simulink model "question2_c"  (R2019b)
settings: Solver=VariableStepAuto  StartTime=0.0  StopTime=10.0  RelTol=1e-3
libraries: fuzblock x50
(part 2 of 2)

== matlab function question2_c/lambda = 10/Subsystem/MATLAB Function ==
  data: A_2 input; y output; A_1 input; A0 input; A1 input; A2 input; B_2 input; B_1 input; B0 input; B1 input; B2 input
function y = fcn(A_2, A_1, A0, A1, A2, B_2, B_1, B0, B1, B2)
u_2_2 = -1;
u_2_1 = -0.7;
u_20 = -0.5;
u_21 = -0.3;
u_22 = 0;

u_1_2 = -0.7;
u_1_1 = -0.4;
u_10 = -0.2;
u_11 = 0;
u_12 = 0.3;

u0_2 = -0.5;
u0_1 = -0.2;
u00 = 0;
u01 = 0.2;
u02 = 0.5;

u1_2 = -0.3;
u1_1 = 0;
u10 = 0.2;
u11 = 0.4;
u12 = 0.7;

u2_2 = 0;
u2_1 = 0.3;
u20 = 0.5;
u21 = 0.7;
u22 = 1;

if ((A0==0) && (A1==0) && (A2==0)) % A_1 ve A_2
    
    if((B0==0) && (B1==0) && (B2==0) && (B_1~= 0) && (B_2~= 0))
        y = A_2*B_2*u_2_2 + A_2*B_1*u_2_1 + A_1*B_1*u_1_1 + A_1*B_2*u_1_2;
    
    elseif((B_2==0) && (B1==0) && (B2==0) && (B_1~= 0) && (B0~= 0))
        y = A_2*B_1*u_2_1 + A_2*B0*u_20 + A_1*B_1*u_1_1 + A_1*B0*u_10;
    
    elseif((B_2==0) && (B_1==0) && (B2==0) && (B0~= 0) && (B1~= 0))
        y = A_2*B0*u_20 + A_2*B1*u_21 + A_1*B0*u_10 + A_1*B1*u_11;
    
    elseif((B0==0) && (B_1==0) && (B_2==0) && (B1~= 0) && (B2~= 0))
        y = A_2*B1*u_21 + A_2*B2*u_22 + A_1*B1*u_11 + A_1*B2*u_12;
    
    elseif((B_1==0) && (B0==0) && (B1==0) && (B2==0))
        y = A_2*B_2*u_2_2 + A_1*B_2*u_1_2;
    
    elseif((B_2==0) && (B0==0) && (B1==0) && (B2==0))
        y = A_2*B_1*u_2_1 + A_1*B_1*u_1_1;
    
    elseif((B_2==0) && (B_1==0) && (B1==0) && (B2==0))
        y = A_2*B0*u_20 + A_1*B0*u_10;
    
    elseif((B_2==0) && (B_1==0) && (B0==0) && (B2==0))
        y = A_2*B1*u_21 + A_1*B1*u_11;
    
    elseif((B_2==0) && (B_1==0) && (B0==0) && (B1==0))
        y = A_2*B2*u_22 + A_1*B2*u_12;
    
    else
        y=0.5;
    end
    
elseif ((A_2==0) && (A1==0) && (A2==0)) % A_1 ve A0
    
    if((B0==0) && (B1==0) && (B2==0) && (B_1~= 0) && (B_2~= 0))
        y = A0*B_2*u0_2 + A0*B_1*u0_1 + A_1*B_1*u_1_1 + A_1*B_2*u_1_2;
    
    elseif((B_2==0) && (B1==0) && (B2==0) && (B_1~= 0) && (B0~= 0))
        y = A0*B_1*u0_1 + A0*B0*u00 + A_1*B_1*u_1_1 + A_1*B0*u_10;
    
    elseif((B_2==0) && (B_1==0) && (B2==0) && (B0~= 0) && (B1~= 0))
        y = A0*B0*u00 + A0*B1*u01 + A_1*B0*u_10 + A_1*B1*u_11;
    
    elseif((B0==0) && (B_1==0) && (B_2==0) && (B1~= 0) && (B2~= 0))
        y = A0*B1*u01 + A0*B2*u02 + A_1*B1*u_11 + A_1*B2*u_12;
    
    elseif((B_1==0) && (B0==0) && (B1==0) && (B2==0))
        y = A0*B_2*u0_2 + A_1*B_2*u_1_2;
    
    elseif((B_2==0) && (B0==0) && (B1==0) && (B2==0))
        y = A0*B_1*u0_1 + A_1*B_1*u_1_1;
    
    elseif((B_2==0) && (B_1==0) && (B1==0) && (B2==0))
        y = A0*B0*u00 + A_1*B0*u_10;
    
    elseif((B_2==0) && (B_1==0) && (B0==0) && (B2==0))
        y = A0*B1*u01 + A_1*B1*u_11;
    
    elseif((B_2==0) && (B_1==0) && (B0==0) && (B1==0))
        y = A0*B2*u02 + A_1*B2*u_12;
    
    else
        y=0.5;
    end
    
elseif ((A_2==0) && (A_1==0) && (A2==0)) % A1 ve A0
    
    if((B0==0) && (B1==0) && (B2==0) && (B_1~= 0) && (B_2~= 0))
        y = A0*B_2*u0_2 + A0*B_1*u0_1 + A1*B_1*u1_1 + A1*B_2*u1_2;
    
    elseif((B_2==0) && (B1==0) && (B2==0) && (B_1~= 0) && (B0~= 0))
        y = A0*B_1*u0_1 + A0*B0*u00 + A1*B_1*u1_1 + A1*B0*u10;
    
    elseif((B_2==0) && (B_1==0) && (B2==0) && (B0~= 0) && (B1~= 0))
        y = A0*B0*u00 + A0*B1*u01 + A1*B0*u10 + A1*B1*u11;
    
    elseif((B0==0) && (B_1==0) && (B_2==0) && (B1~= 0) && (B2~= 0))
        y = A0*B1*u01 + A0*B2*u02 + A1*B1*u11 + A1*B2*u12;
    
    elseif((B_1==0) && (B0==0) && (B1==0) && (B2==0))
        y = A0*B_2*u0_2 + A1*B_2*u1_2;
    
    elseif((B_2==0) && (B0==0) && (B1==0) && (B2==0))
        y = A0*B_1*u0_1 + A1*B_1*u1_1;
    
    elseif((B_2==0) && (B_1==0) && (B1==0) && (B2==0))
        y = A0*B0*u00 + A1*B0*u10;
    
    elseif((B_2==0) && (B_1==0) && (B0==0) && (B2==0))
        y = A0*B1*u01 + A1*B1*u11;
    
    elseif((B_2==0) && (B_1==0) && (B0==0) && (B1==0))
        y = A0*B2*u02 + A1*B2*u12;
    
    else
        y=0.5;
    end
    
elseif ((A_2==0) && (A_1==0) && (A0==0)) % A1 ve A2
    
    if((B0==0) && (B1==0) && (B2==0) && (B_1~= 0) && (B_2~= 0))
        y = A2*B_2*u2_2 + A2*B_1*u2_1 + A1*B_1*u1_1 + A1*B_2*u1_2;
    
    elseif((B_2==0) && (B1==0) && (B2==0) && (B_1~= 0) && (B0~= 0))
        y = A2*B_1*u2_1 + A2*B0*u20 + A1*B_1*u1_1 + A1*B0*u10;
    
    elseif((B_2==0) && (B_1==0) && (B2==0) && (B0~= 0) && (B1~= 0))
        y = A2*B0*u20 + A2*B1*u21 + A1*B0*u10 + A1*B1*u11;
    
    elseif((B0==0) && (B_1==0) && (B_2==0) && (B1~= 0) && (B2~= 0))
        y = A2*B1*u21 + A2*B2*u22 + A1*B1*u11 + A1*B2*u12;
    
    elseif((B_1==0) && (B0==0) && (B1==0) && (B2==0))
        y = A2*B_2*u2_2 + A1*B_2*u1_2;
    
    elseif((B_2==0) && (B0==0) && (B1==0) && (B2==0))
        y = A2*B_1*u2_1 + A1*B_1*u1_1;
    
    elseif((B_2==0) && (B_1==0) && (B1==0) && (B2==0))
        y = A2*B0*u20 + A1*B0*u10;
    
    elseif((B_2==0) && (B_1==0) && (B0==0) && (B2==0))
        y = A2*B1*u21 + A1*B1*u11;
    
    elseif((B_2==0) && (B_1==0) && (B0==0) && (B1==0))
        y = A2*B2*u22 + A1*B2*u12;
    
    else
        y=0.5;
    end
else
    y=0.5;
end

== matlab function question2_c/lambda = 100/CSTR System/MATLAB Function ==
  data: x1 input; x1 output; x2 input; x3 input; v1 input; x2 output; x3 output
% Runge Kutta method for CSTR 
% Da1, Da2, Da3, d2 are CSTR parameters
% v1 is control input.
% h is the sampling time.
% x1, x2, x3 are the states of the system.

function  [x1,x2,x3]=CSTR_runga_kutta_new(x1,x2,x3,v1)
Da1 = 3; Da2 = 0.5; Da3 = 1; d2 = 1; h = 0.1;

k1x1=1-x1-Da1*x1+Da2*x2*x2;
k1x2=-x2+Da1*x1-Da2*x2*x2-Da3*d2*x2*x2+v1;
k1x3=-x3+Da3*d2*x2*x2;



k2x1=1-(x1+h*k1x1/2)-Da1*(x1+h*k1x1/2)+Da2*(x2+h*k1x2/2)*(x2+h*k1x2/2);
k2x2=-(x2+h*k1x2/2)+Da1*(x1+h*k1x1/2)-Da2*(x2+h*k1x2/2)*(x2+h*k1x2/2)-Da3*d2*(x2+h*k1x2/2)*(x2+h*k1x2/2)+v1;
k2x3=-(x3+h*k1x3/2 )+Da3*d2*(x2+h*k1x2/2)*(x2+h*k1x2/2);


k3x1=1-(x1+h*k2x1/2)-Da1*(x1+h*k2x1/2)+Da2*(x2+h*k2x2/2)*(x2+h*k2x2/2);
k3x2=-(x2+h*k2x2/2)+Da1*(x1+h*k2x1/2)-Da2*(x2+h*k2x2/2)*(x2+h*k2x2/2)-Da3*d2*(x2+h*k2x2/2)*(x2+h*k2x2/2)+v1;
k3x3=-(x3+h*k2x3/2)+Da3*d2*(x2+h*k2x2/2)*(x2+h*k2x2/2);



k4x1=1-(x1+h*k3x1)-Da1*(x1+h*k3x1)+Da2*(x2+h*k3x2)*(x2+h*k3x2);
k4x2=-(x2+h*k3x2)+Da1*(x1+h*k3x1)-Da2*(x2+h*k3x2)*(x2+h*k3x2)-Da3*d2*(x2+h*k3x2)*(x2+h*k3x2)+v1;
k4x3=-(x3+h*k3x3)+Da3*d2*(x2+h*k3x2)*(x2+h*k3x2);



x1=x1+(h/6)*(k1x1+2*k2x1+2*k3x1+k4x1);
x2=x2+(h/6)*(k1x2+2*k2x2+2*k3x2+k4x2);
x3=x3+(h/6)*(k1x3+2*k2x3+2*k3x3+k4x3);

== matlab function question2_c/lambda = 100/Subsystem/MATLAB Function ==
  data: A_2 input; y output; A_1 input; A0 input; A1 input; A2 input; B_2 input; B_1 input; B0 input; B1 input; B2 input
function y = fcn(A_2, A_1, A0, A1, A2, B_2, B_1, B0, B1, B2)
u_2_2 = -1;
u_2_1 = -0.7;
u_20 = -0.5;
u_21 = -0.3;
u_22 = 0;

u_1_2 = -0.7;
u_1_1 = -0.4;
u_10 = -0.2;
u_11 = 0;
u_12 = 0.3;

u0_2 = -0.5;
u0_1 = -0.2;
u00 = 0;
u01 = 0.2;
u02 = 0.5;

u1_2 = -0.3;
u1_1 = 0;
u10 = 0.2;
u11 = 0.4;
u12 = 0.7;

u2_2 = 0;
u2_1 = 0.3;
u20 = 0.5;
u21 = 0.7;
u22 = 1;

if ((A0==0) && (A1==0) && (A2==0)) % A_1 ve A_2
    
    if((B0==0) && (B1==0) && (B2==0) && (B_1~= 0) && (B_2~= 0))
        y = A_2*B_2*u_2_2 + A_2*B_1*u_2_1 + A_1*B_1*u_1_1 + A_1*B_2*u_1_2;
    
    elseif((B_2==0) && (B1==0) && (B2==0) && (B_1~= 0) && (B0~= 0))
        y = A_2*B_1*u_2_1 + A_2*B0*u_20 + A_1*B_1*u_1_1 + A_1*B0*u_10;
    
    elseif((B_2==0) && (B_1==0) && (B2==0) && (B0~= 0) && (B1~= 0))
        y = A_2*B0*u_20 + A_2*B1*u_21 + A_1*B0*u_10 + A_1*B1*u_11;
    
    elseif((B0==0) && (B_1==0) && (B_2==0) && (B1~= 0) && (B2~= 0))
        y = A_2*B1*u_21 + A_2*B2*u_22 + A_1*B1*u_11 + A_1*B2*u_12;
    
    elseif((B_1==0) && (B0==0) && (B1==0) && (B2==0))
        y = A_2*B_2*u_2_2 + A_1*B_2*u_1_2;
    
    elseif((B_2==0) && (B0==0) && (B1==0) && (B2==0))
        y = A_2*B_1*u_2_1 + A_1*B_1*u_1_1;
    
    elseif((B_2==0) && (B_1==0) && (B1==0) && (B2==0))
        y = A_2*B0*u_20 + A_1*B0*u_10;
    
    elseif((B_2==0) && (B_1==0) && (B0==0) && (B2==0))
        y = A_2*B1*u_21 + A_1*B1*u_11;
    
    elseif((B_2==0) && (B_1==0) && (B0==0) && (B1==0))
        y = A_2*B2*u_22 + A_1*B2*u_12;
    
    else
        y=0.5;
    end
    
elseif ((A_2==0) && (A1==0) && (A2==0)) % A_1 ve A0
    
    if((B0==0) && (B1==0) && (B2==0) && (B_1~= 0) && (B_2~= 0))
        y = A0*B_2*u0_2 + A0*B_1*u0_1 + A_1*B_1*u_1_1 + A_1*B_2*u_1_2;
    
    elseif((B_2==0) && (B1==0) && (B2==0) && (B_1~= 0) && (B0~= 0))
        y = A0*B_1*u0_1 + A0*B0*u00 + A_1*B_1*u_1_1 + A_1*B0*u_10;
    
    elseif((B_2==0) && (B_1==0) && (B2==0) && (B0~= 0) && (B1~= 0))
        y = A0*B0*u00 + A0*B1*u01 + A_1*B0*u_10 + A_1*B1*u_11;
    
    elseif((B0==0) && (B_1==0) && (B_2==0) && (B1~= 0) && (B2~= 0))
        y = A0*B1*u01 + A0*B2*u02 + A_1*B1*u_11 + A_1*B2*u_12;
    
    elseif((B_1==0) && (B0==0) && (B1==0) && (B2==0))
        y = A0*B_2*u0_2 + A_1*B_2*u_1_2;
    
    elseif((B_2==0) && (B0==0) && (B1==0) && (B2==0))
        y = A0*B_1*u0_1 + A_1*B_1*u_1_1;
    
    elseif((B_2==0) && (B_1==0) && (B1==0) && (B2==0))
        y = A0*B0*u00 + A_1*B0*u_10;
    
    elseif((B_2==0) && (B_1==0) && (B0==0) && (B2==0))
        y = A0*B1*u01 + A_1*B1*u_11;
    
    elseif((B_2==0) && (B_1==0) && (B0==0) && (B1==0))
        y = A0*B2*u02 + A_1*B2*u_12;
    
    else
        y=0.5;
    end
    
elseif ((A_2==0) && (A_1==0) && (A2==0)) % A1 ve A0
    
    if((B0==0) && (B1==0) && (B2==0) && (B_1~= 0) && (B_2~= 0))
        y = A0*B_2*u0_2 + A0*B_1*u0_1 + A1*B_1*u1_1 + A1*B_2*u1_2;
    
    elseif((B_2==0) && (B1==0) && (B2==0) && (B_1~= 0) && (B0~= 0))
        y = A0*B_1*u0_1 + A0*B0*u00 + A1*B_1*u1_1 + A1*B0*u10;
    
    elseif((B_2==0) && (B_1==0) && (B2==0) && (B0~= 0) && (B1~= 0))
        y = A0*B0*u00 + A0*B1*u01 + A1*B0*u10 + A1*B1*u11;
    
    elseif((B0==0) && (B_1==0) && (B_2==0) && (B1~= 0) && (B2~= 0))
        y = A0*B1*u01 + A0*B2*u02 + A1*B1*u11 + A1*B2*u12;
    
    elseif((B_1==0) && (B0==0) && (B1==0) && (B2==0))
        y = A0*B_2*u0_2 + A1*B_2*u1_2;
    
    elseif((B_2==0) && (B0==0) && (B1==0) && (B2==0))
        y = A0*B_1*u0_1 + A1*B_1*u1_1;
    
    elseif((B_2==0) && (B_1==0) && (B1==0) && (B2==0))
        y = A0*B0*u00 + A1*B0*u10;
    
    elseif((B_2==0) && (B_1==0) && (B0==0) && (B2==0))
        y = A0*B1*u01 + A1*B1*u11;
    
    elseif((B_2==0) && (B_1==0) && (B0==0) && (B1==0))
        y = A0*B2*u02 + A1*B2*u12;
    
    else
        y=0.5;
    end
    
elseif ((A_2==0) && (A_1==0) && (A0==0)) % A1 ve A2
    
    if((B0==0) && (B1==0) && (B2==0) && (B_1~= 0) && (B_2~= 0))
        y = A2*B_2*u2_2 + A2*B_1*u2_1 + A1*B_1*u1_1 + A1*B_2*u1_2;
    
    elseif((B_2==0) && (B1==0) && (B2==0) && (B_1~= 0) && (B0~= 0))
        y = A2*B_1*u2_1 + A2*B0*u20 + A1*B_1*u1_1 + A1*B0*u10;
    
    elseif((B_2==0) && (B_1==0) && (B2==0) && (B0~= 0) && (B1~= 0))
        y = A2*B0*u20 + A2*B1*u21 + A1*B0*u10 + A1*B1*u11;
    
    elseif((B0==0) && (B_1==0) && (B_2==0) && (B1~= 0) && (B2~= 0))
        y = A2*B1*u21 + A2*B2*u22 + A1*B1*u11 + A1*B2*u12;
    
    elseif((B_1==0) && (B0==0) && (B1==0) && (B2==0))
        y = A2*B_2*u2_2 + A1*B_2*u1_2;
    
    elseif((B_2==0) && (B0==0) && (B1==0) && (B2==0))
        y = A2*B_1*u2_1 + A1*B_1*u1_1;
    
    elseif((B_2==0) && (B_1==0) && (B1==0) && (B2==0))
        y = A2*B0*u20 + A1*B0*u10;
    
    elseif((B_2==0) && (B_1==0) && (B0==0) && (B2==0))
        y = A2*B1*u21 + A1*B1*u11;
    
    elseif((B_2==0) && (B_1==0) && (B0==0) && (B1==0))
        y = A2*B2*u22 + A1*B2*u12;
    
    else
        y=0.5;
    end
else
    y=0.5;
end
